simulink model "niof_model"  (R2021a)
settings: Solver=ode23tb  StartTime=0.0  StopTime=2  RelTol=1e-3
values from neighbouring files (symbols this model uses):
  h0 = ds.DateTime(1).Hour + ds.DateTime(1).Minute/60    [compiler_niof_model.m]
  S_area_hole = 0.01    [set_params_blocks.m]
undefined symbols (not defined in the file or in its folder): crop_GH1_NFT_slot1___C, crop_GH1_NFT_slot1___N, crop_GH1_NFT_slot1___R, crop_GH1_NFT_slot2___C, crop_GH1_NFT_slot2___N, crop_GH1_NFT_slot2___R, crop_GH1_NFT_slot3___C, crop_GH1_NFT_slot3___N, crop_GH1_NFT_slot3___R, crop_GH1_NFT_slot4___C, crop_GH1_NFT_slot4___N, crop_GH1_NFT_slot4___R, crop_GH1_RF_slot1___C, crop_GH1_RF_slot1___N, crop_GH1_RF_slot1___R, crop_GH1_RF_slot2___C, crop_GH1_RF_slot2___N, crop_GH1_RF_slot2___R, crop_GH1_RF_slot3___C, crop_GH1_RF_slot3___N, crop_GH1_RF_slot3___R, crop_GH1_RF_slot4___C, crop_GH1_RF_slot4___N, crop_GH1_RF_slot4___R, crop_GH2_RF_slot1___C, crop_GH2_RF_slot1___N, crop_GH2_RF_slot1___R, crop_GH2_RF_slot2___C, crop_GH2_RF_slot2___N, crop_GH2_RF_slot2___R, crop_GH2_RF_slot3___C, crop_GH2_RF_slot3___N, crop_GH2_RF_slot3___R, crop_GH2_RF_slot4___C, crop_GH2_RF_slot4___N, crop_GH2_RF_slot4___R, crop_GH2_TRAD_slot1___C, crop_GH2_TRAD_slot1___N, crop_GH2_TRAD_slot1___R, crop_GH2_TRAD_slot2___C, crop_GH2_TRAD_slot2___N, crop_GH2_TRAD_slot2___R, crop_GH2_TRAD_slot3___C, crop_GH2_TRAD_slot3___N, crop_GH2_TRAD_slot3___R, crop_GH2_TRAD_slot4___C, crop_GH2_TRAD_slot4___N, crop_GH2_TRAD_slot4___R, fish, GH3_Tank1_tend, GH3_Tank2_tend, GH3_Tank3_tend, GH3_Tank4_tend, tp_biofilter___T, tp_fish_C___T, tp_fish_M___T, tp_fish_S___T, tp_fish_T___T, tp_GH1_bio___T, tp_GH1_NFT___T ... (+3)
libraries: HORTISIM x152
(part 3 of 4)

== system niof_model/GH1/NFT System/Control 1 ==
  Crop : Inport
  Prune Policy : HORTISIM/Horticulture/Controls/Prune Policy  SystemSampleTime=-1  VariantActivationTime=update diagram  Latency=0  AutoFrameSizeCalculation=off
      settings: SourceProductName=Horti Simulator
  Scalar2Bus Control Crop : HORTISIM/Other  Functions/Scalar2Bus Control Crop  SystemSampleTime=-1  VariantActivationTime=update diagram  Latency=0  AutoFrameSizeCalculation=off
      settings: SourceProductName=Horti Simulator
  Start/Stop Window : HORTISIM/Other  Functions/Start//Stop Window  tinit=GH1_NFTSystem_Control1_tinit  tend=GH1_NFTSystem_Control1_tend
      settings: SourceProductName=Horti Simulator
  CC : Outport
  wires:
  ? -> Scalar2Bus Control Crop/3
  Prune Policy/1 -> Scalar2Bus Control Crop/1
  ? -> Scalar2Bus Control Crop/2
  Scalar2Bus Control Crop/1 -> CC/1
  Start/Stop Window/1 -> Scalar2Bus Control Crop/4
  Crop/1 -> Prune Policy/1

== system niof_model/GH1/NFT System/Control 2 ==
  Crop : Inport
  Prune Policy : HORTISIM/Horticulture/Controls/Prune Policy  SystemSampleTime=-1  VariantActivationTime=update diagram  Latency=0  AutoFrameSizeCalculation=off
      settings: SourceProductName=Horti Simulator
  Scalar2Bus Control Crop : HORTISIM/Other  Functions/Scalar2Bus Control Crop  SystemSampleTime=-1  VariantActivationTime=update diagram  Latency=0  AutoFrameSizeCalculation=off
      settings: SourceProductName=Horti Simulator
  Start/Stop Window : HORTISIM/Other  Functions/Start//Stop Window  tinit=GH1_NFTSystem_Control2_tinit  tend=GH1_NFTSystem_Control2_tend
      settings: SourceProductName=Horti Simulator
  CC : Outport
  wires:
  ? -> Scalar2Bus Control Crop/3
  Prune Policy/1 -> Scalar2Bus Control Crop/1
  ? -> Scalar2Bus Control Crop/2
  Scalar2Bus Control Crop/1 -> CC/1
  Start/Stop Window/1 -> Scalar2Bus Control Crop/4
  Crop/1 -> Prune Policy/1

== system niof_model/GH1/NFT System/Control 3 ==
  Crop : Inport
  Prune Policy : HORTISIM/Horticulture/Controls/Prune Policy  SystemSampleTime=-1  VariantActivationTime=update diagram  Latency=0  AutoFrameSizeCalculation=off
      settings: SourceProductName=Horti Simulator
  Scalar2Bus Control Crop : HORTISIM/Other  Functions/Scalar2Bus Control Crop  SystemSampleTime=-1  VariantActivationTime=update diagram  Latency=0  AutoFrameSizeCalculation=off
      settings: SourceProductName=Horti Simulator
  Start/Stop Window : HORTISIM/Other  Functions/Start//Stop Window  tinit=GH1_NFTSystem_Control3_tinit  tend=GH1_NFTSystem_Control3_tend
      settings: SourceProductName=Horti Simulator
  CC : Outport
  wires:
  ? -> Scalar2Bus Control Crop/3
  Prune Policy/1 -> Scalar2Bus Control Crop/1
  ? -> Scalar2Bus Control Crop/2
  Scalar2Bus Control Crop/1 -> CC/1
  Start/Stop Window/1 -> Scalar2Bus Control Crop/4
  Crop/1 -> Prune Policy/1

== system niof_model/GH1/NFT System/Control 4 ==
  Crop : Inport
  Prune Policy : HORTISIM/Horticulture/Controls/Prune Policy  SystemSampleTime=-1  VariantActivationTime=update diagram  Latency=0  AutoFrameSizeCalculation=off
      settings: SourceProductName=Horti Simulator
  Scalar2Bus Control Crop : HORTISIM/Other  Functions/Scalar2Bus Control Crop  SystemSampleTime=-1  VariantActivationTime=update diagram  Latency=0  AutoFrameSizeCalculation=off
      settings: SourceProductName=Horti Simulator
  Start/Stop Window : HORTISIM/Other  Functions/Start//Stop Window  tinit=GH1_NFTSystem_Control4_tinit  tend=GH1_NFTSystem_Control4_tend
      settings: SourceProductName=Horti Simulator
  CC : Outport
  wires:
  ? -> Scalar2Bus Control Crop/3
  Prune Policy/1 -> Scalar2Bus Control Crop/1
  ? -> Scalar2Bus Control Crop/2
  Scalar2Bus Control Crop/1 -> CC/1
  Start/Stop Window/1 -> Scalar2Bus Control Crop/4
  Crop/1 -> Prune Policy/1

== system niof_model/GH1/NFT System/Reorder signals ==
  In Bus Element : Inport  PortName=C1  Element=Crop
  In Bus Element1 : Inport  PortName=C1  Element=Crop1
  In Bus Element2 : Inport  PortName=C1  Element=Crop2
  In Bus Element3 : Inport  PortName=C1  Element=Crop3
  WT : Inport  Port=2
  Subsystem : Subsystem
      settings: PortSchema="{\"entries\":[{\"content\":{\"sides\":[{\"content\":{\"connectorIds\":[]},\"type\":\"ConnectorPlacement.EquallySpacedRectSide\",\"uuid\":\"331b7e07-99e0-48a1-afa9-efd959d86c3c\"},{\"content\":{\"connectorIds\":[\"Out1\",\"Out2\"],\"side\":\"RIGHT\"},\"type\":\"ConnectorPlacement.EquallySpacedRectSide\",\"uuid\":\"88f560c2-c33d-415c-abbb-9cce13a50e34\"},{\"content\":{\"connectorIds\":[\"In1\",\"In2\",\"In3\",\"In4\"],\"side\":\"TOP\"},\"type\":\"ConnectorPlacement.EquallySpacedRectSide\",\"uuid\":\"5809bd20-6d1a-4a08-a3be-af6196f2651a\"},{\"content\":{\"connectorIds\":[],\"side\":\"BOTTOM\"},\"type\":\"ConnectorPlacement.EquallySpacedRectSide\",\"uuid\":\"0451beb0-e3d9-4028-a291-a4662efcb901\"}]},\"type\":\"ConnectorPlacement.EquallySpacedConnector\",\"uuid\":\"8352e301-80a0-449c-83b8-038a5d79df4c\"}],\"packageUris\":[\"http://schema.mathworks.com/mf0/Connector/R2020b\"],\"version\":\"1.0\"}"
  Subsystem1 : Subsystem
      settings: PortSchema="{\"entries\":[{\"content\":{\"sides\":[{\"content\":{\"connectorIds\":[\"In1\",\"In2\",\"In3\",\"In4\"]},\"type\":\"ConnectorPlacement.EquallySpacedRectSide\",\"uuid\":\"4fbee580-d560-4e1c-bbb5-c1692f8814f1\"},{\"content\":{\"connectorIds\":[\"Out1\",\"Out2\",\"Out3\",\"Out4\"],\"side\":\"RIGHT\"},\"type\":\"ConnectorPlacement.EquallySpacedRectSide\",\"uuid\":\"81a4a23d-0981-460c-8110-0a6c3dae9561\"},{\"content\":{\"connectorIds\":[\"In5\"],\"side\":\"TOP\"},\"type\":\"ConnectorPlacement.EquallySpacedRectSide\",\"uuid\":\"d86bf355-ad16-490c-942f-99534b60638b\"},{\"content\":{\"connectorIds\":[\"Out5\"],\"side\":\"BOTTOM\"},\"type\":\"ConnectorPlacement.EquallySpacedRectSide\",\"uuid\":\"eaa009ab-e9b5-48b4-8c60-43d182c3bfd7\"}]},\"type\":\"ConnectorPlacement.EquallySpacedConnector\",\"uuid\":\"d99c9aa8-04cd-4090-9f71-30da2befe22b\"}],\"packageUris\":[\"http://schema.mathworks.com/mf0/Connector/R2020b\"],\"version\":\"1.0\"}"
  Out Bus Element : Outport  PortName=Subs  Element=Subs1
  Out Bus Element1 : Outport  PortName=Subs  Element=Subs2
  Out Bus Element2 : Outport  PortName=Subs  Element=Subs3
  Out Bus Element3 : Outport  PortName=Subs  Element=Subs4
  CropInt : Outport  Port=2
  fout : Outport  Port=3
  R : Outport  Port=4
  wires:
  WT/1 -> Subsystem1/5(WT)
  Subsystem1/4(Subs4) -> Out Bus Element3/1
  In Bus Element2/1 -> Subsystem/3(Crop2), Subsystem1/2(C2)
  Subsystem1/3(Subs3) -> Out Bus Element2/1
  In Bus Element/1 -> Subsystem1/1(C1), Subsystem/4(Crop1)
  Subsystem1/1(Subs) -> Out Bus Element/1
  Subsystem1/2(Subs2) -> Out Bus Element1/1
  Subsystem/2(Out2) -> R/1
  In Bus Element3/1 -> Subsystem1/3(C3), Subsystem/1(Crop3)
  Subsystem/1(Out1) -> fout/1
  In Bus Element1/1 -> Subsystem1/4(C4), Subsystem/2(Crop4)
  Subsystem1/5(Out3) -> CropInt/1

== system niof_model/GH1/RF System/Control 1 ==
  Crop : Inport
  Prune Policy : HORTISIM/Horticulture/Controls/Prune Policy  SystemSampleTime=-1  VariantActivationTime=update diagram  Latency=0  AutoFrameSizeCalculation=off
      settings: SourceProductName=Horti Simulator
  Scalar2Bus Control Crop : HORTISIM/Other  Functions/Scalar2Bus Control Crop  SystemSampleTime=-1  VariantActivationTime=update diagram  Latency=0  AutoFrameSizeCalculation=off
      settings: SourceProductName=Horti Simulator
  Start/Stop Window : HORTISIM/Other  Functions/Start//Stop Window  tinit=GH1_RFSystem_Control1_tinit  tend=GH1_RFSystem_Control1_tend
      settings: SourceProductName=Horti Simulator
  CC : Outport
  wires:
  ? -> Scalar2Bus Control Crop/3
  Prune Policy/1 -> Scalar2Bus Control Crop/1
  ? -> Scalar2Bus Control Crop/2
  Scalar2Bus Control Crop/1 -> CC/1
  Start/Stop Window/1 -> Scalar2Bus Control Crop/4
  Crop/1 -> Prune Policy/1

== system niof_model/GH1/RF System/Control 2 ==
  Crop : Inport
  Prune Policy : HORTISIM/Horticulture/Controls/Prune Policy  SystemSampleTime=-1  VariantActivationTime=update diagram  Latency=0  AutoFrameSizeCalculation=off
      settings: SourceProductName=Horti Simulator
  Scalar2Bus Control Crop : HORTISIM/Other  Functions/Scalar2Bus Control Crop  SystemSampleTime=-1  VariantActivationTime=update diagram  Latency=0  AutoFrameSizeCalculation=off
      settings: SourceProductName=Horti Simulator
  Start/Stop Window : HORTISIM/Other  Functions/Start//Stop Window  tinit=GH1_RFSystem_Control2_tinit  tend=GH1_RFSystem_Control2_tend
      settings: SourceProductName=Horti Simulator
  CC : Outport
  wires:
  ? -> Scalar2Bus Control Crop/3
  Prune Policy/1 -> Scalar2Bus Control Crop/1
  ? -> Scalar2Bus Control Crop/2
  Scalar2Bus Control Crop/1 -> CC/1
  Start/Stop Window/1 -> Scalar2Bus Control Crop/4
  Crop/1 -> Prune Policy/1

== system niof_model/GH1/RF System/Control 3 ==
  Crop : Inport
  Prune Policy : HORTISIM/Horticulture/Controls/Prune Policy  SystemSampleTime=-1  VariantActivationTime=update diagram  Latency=0  AutoFrameSizeCalculation=off
      settings: SourceProductName=Horti Simulator
  Scalar2Bus Control Crop : HORTISIM/Other  Functions/Scalar2Bus Control Crop  SystemSampleTime=-1  VariantActivationTime=update diagram  Latency=0  AutoFrameSizeCalculation=off
      settings: SourceProductName=Horti Simulator
  Start/Stop Window : HORTISIM/Other  Functions/Start//Stop Window  tinit=GH1_RFSystem_Control3_tinit  tend=GH1_RFSystem_Control3_tend
      settings: SourceProductName=Horti Simulator
  CC : Outport
  wires:
  ? -> Scalar2Bus Control Crop/3
  Prune Policy/1 -> Scalar2Bus Control Crop/1
  ? -> Scalar2Bus Control Crop/2
  Scalar2Bus Control Crop/1 -> CC/1
  Start/Stop Window/1 -> Scalar2Bus Control Crop/4
  Crop/1 -> Prune Policy/1

== system niof_model/GH1/RF System/Control 4 ==
  Crop : Inport
  Prune Policy : HORTISIM/Horticulture/Controls/Prune Policy  SystemSampleTime=-1  VariantActivationTime=update diagram  Latency=0  AutoFrameSizeCalculation=off
      settings: SourceProductName=Horti Simulator
  Scalar2Bus Control Crop : HORTISIM/Other  Functions/Scalar2Bus Control Crop  SystemSampleTime=-1  VariantActivationTime=update diagram  Latency=0  AutoFrameSizeCalculation=off
      settings: SourceProductName=Horti Simulator
  Start/Stop Window : HORTISIM/Other  Functions/Start//Stop Window  tinit=GH1_RFSystem_Control4_tinit  tend=GH1_RFSystem_Control4_tend
      settings: SourceProductName=Horti Simulator
  CC : Outport
  wires:
  ? -> Scalar2Bus Control Crop/3
  Prune Policy/1 -> Scalar2Bus Control Crop/1
  ? -> Scalar2Bus Control Crop/2
  Scalar2Bus Control Crop/1 -> CC/1
  Start/Stop Window/1 -> Scalar2Bus Control Crop/4
  Crop/1 -> Prune Policy/1

== system niof_model/GH1/RF System/Subsystem ==
  Crop2 : Inport
  Crop1 : Inport  Port=2
  Crop3 : Inport  Port=3
  Crop4 : Inport  Port=4
  CropToTank Parser{1..4} (4 alike) : HORTISIM/Other  Functions/CropToTank Parser  SystemSampleTime=-1  VariantActivationTime=update diagram  Latency=0  AutoFrameSizeCalculation=off
      settings: SourceProductName=Horti Simulator
  Vector Concatenate : Concatenate  NumInputs=4  Mode=Multidimensional array
  Vector Concatenate1 : Concatenate  NumInputs=4  Mode=Multidimensional array  ConcatenateDimension=2
  Out1 : Outport
  Out2 : Outport  Port=2
  wires:
  Crop2/1 -> CropToTank Parser2/1
  CropToTank Parser2/2 -> Vector Concatenate1/2
  CropToTank Parser1/2 -> Vector Concatenate1/1
  Vector Concatenate1/1 -> Out2/1
  Vector Concatenate/1 -> Out1/1
  Crop1/1 -> CropToTank Parser1/1
  CropToTank Parser2/1 -> Vector Concatenate/2
  CropToTank Parser1/1 -> Vector Concatenate/1
  Crop3/1 -> CropToTank Parser3/1
  CropToTank Parser3/1 -> Vector Concatenate/3
  Crop4/1 -> CropToTank Parser4/1
  CropToTank Parser4/1 -> Vector Concatenate/4
  CropToTank Parser3/2 -> Vector Concatenate1/3
  CropToTank Parser4/2 -> Vector Concatenate1/4

== system niof_model/GH1/RF System/Subsystem1 ==
  In Bus Element : Inport  PortName=C1  Element=Crop
  In Bus Element1 : Inport  PortName=C1  Element=Crop1
  In Bus Element2 : Inport  PortName=C1  Element=Crop2
  In Bus Element3 : Inport  PortName=C1  Element=Crop3
  WT : Inport  Port=2
  Crop Interactio with Climate : Subsystem
  TankToCrop Parser Several : Subsystem
      settings: PortSchema="{\"entries\":[{\"content\":{\"sides\":[{\"content\":{\"connectorIds\":[\"In1\",\"In2\",\"In3\",\"In4\"]},\"type\":\"ConnectorPlacement.EquallySpacedRectSide\",\"uuid\":\"99f6f79d-93b3-4d94-9532-d82544948055\"},{\"content\":{\"connectorIds\":[\"Out1\",\"Out2\",\"Out3\",\"Out4\"],\"side\":\"RIGHT\"},\"type\":\"ConnectorPlacement.EquallySpacedRectSide\",\"uuid\":\"ca15eaf2-1366-4114-b322-5e88a02c6d72\"},{\"content\":{\"connectorIds\":[\"In5\"],\"side\":\"TOP\"},\"type\":\"ConnectorPlacement.EquallySpacedRectSide\",\"uuid\":\"2404a174-e0a1-432d-a5bc-62127522feaf\"}]},\"type\":\"ConnectorPlacement.EquallySpacedConnector\",\"uuid\":\"a404298f-e4a9-4dc3-b790-516f41057283\"}],\"packageUris\":[\"http://schema.mathworks.com/mf0/Connector/R2020b\"],\"version\":\"1.0\"}"
  Subs1 : Outport
  Subs2 : Outport  Port=2
  Subs3 : Outport  Port=3
  Subs4 : Outport  Port=4
  Out3 : Outport  Port=5
  wires:
  Crop Interactio with Climate/1(OutBus) -> Out3/1
  WT/1 -> TankToCrop Parser Several/5(WT)
  TankToCrop Parser Several/1(Subs1) -> Subs1/1
  In Bus Element3/1 -> Crop Interactio with Climate/4(C4), TankToCrop Parser Several/4(C4)
  TankToCrop Parser Several/3(Subs3) -> Subs3/1
  TankToCrop Parser Several/4(Subs4) -> Subs4/1
  TankToCrop Parser Several/2(Subs2) -> Subs2/1
  In Bus Element2/1 -> Crop Interactio with Climate/3(C3), TankToCrop Parser Several/3(C3)
  In Bus Element/1 -> Crop Interactio with Climate/1(C1), TankToCrop Parser Several/1(C1)
  In Bus Element1/1 -> Crop Interactio with Climate/2(C2), TankToCrop Parser Several/2(C2)

== system niof_model/GH1/Subsystem1/Subsystem3 ==
  In1 : Inport
  In2 : Inport  Port=2
  Abs : Abs  ZeroCross=off
  Bus Creator : BusCreator  Inputs=3  OutDataTypeStr=Bus: FLOW  NonVirtualBus=on
  Bus Selector : BusSelector  OutputSignals=f
  Bus Selector1 : BusSelector  OutputSignals=f
  If : If  IfExpression=u1 <1e-8  ZeroCross=off
  If Action Subsystem : Subsystem  TreatAsAtomicUnit=on
  If Action Subsystem1 : Subsystem  TreatAsAtomicUnit=on
  Merge : Merge
  Merge1 : Merge
  Merge2 : Merge
  Sum : Sum  Inputs=|++
  Out1 : Outport
  wires:
  In1/1 -> [F1], Bus Selector/1
  In2/1 -> [F2], Bus Selector1/1
  Bus Selector/1 -> [f1]  "<f>"
  Bus Selector1/1 -> [f2]  "<f>"
  [f1] -> Sum/1
  [f2] -> Sum/2
  Sum/1 -> Abs/1
  Abs/1 -> If/1
  If/1 -> If Action Subsystem/Action
  [F1] -> If Action Subsystem/1(In1)
  [F2] -> If Action Subsystem1/2(In2)
  [F1] -> If Action Subsystem1/1(In1)
  Bus Creator/1 -> Out1/1
  If Action Subsystem1/3(X) -> Merge2/2
  If Action Subsystem/3(X) -> Merge2/1
  If Action Subsystem1/2(T) -> Merge1/2
  If Action Subsystem/2(T) -> Merge1/1
  If Action Subsystem1/1(f) -> Merge/2
  If Action Subsystem/1(f) -> Merge/1
  Merge/1 -> Bus Creator/1  "f"
  Merge1/1 -> Bus Creator/2  "T"
  Merge2/1 -> Bus Creator/3  "X"
  If/2 -> If Action Subsystem1/Action

== system niof_model/GH2/Mezcla Calor, Vapor de agua y CO2 desde los tanques de agua y la plantación/Crop2ExtArray ==
  In1 : Inport
  Bus Selector : BusSelector  OutputSignals=HeatVars.QV,HeatVars.QT,A_v,CC
  Scope : Scope
  Vector Concatenate : Concatenate  NumInputs=4  Mode=Multidimensional array
  Out1 : Outport
  wires:
  Vector Concatenate/1 -> Out1/1
  Bus Selector/4 -> Vector Concatenate/4  "<CC>"
  Bus Selector/3 -> Vector Concatenate/3  "<A_v>"
  Bus Selector/2 -> Scope/1, Vector Concatenate/2  "<QT>"
  Bus Selector/1 -> Vector Concatenate/1  "<QV>"
  In1/1 -> Bus Selector/1

== system niof_model/GH2/Mezcla Calor, Vapor de agua y CO2 desde los tanques de agua y la plantación/MatrixExt2Bus ==
  In1 : Inport
  Demux : Demux
  "Scalar2Bus Ext Signal " : HORTISIM/Other  Functions/Scalar2Bus Ext Signal    SystemSampleTime=-1  VariantActivationTime=update diagram  Latency=0  AutoFrameSizeCalculation=off
      settings: SourceProductName=Horti Simulator
  Scope : Scope
  Scope1 : Scope
  Sum of Elements : Sum  Inputs=+  CollapseMode=Specified dimension  CollapseDim=2
  CoCl : Outport
  wires:
  "Scalar2Bus Ext Signal "/1 -> CoCl/1
  Demux/4 -> "Scalar2Bus Ext Signal "/4
  Demux/3 -> Scope1/1, "Scalar2Bus Ext Signal "/3
  Demux/2 -> Scope/1, "Scalar2Bus Ext Signal "/2
  Demux/1 -> "Scalar2Bus Ext Signal "/1
  Sum of Elements/1 -> Demux/1
  In1/1 -> Sum of Elements/1

== system niof_model/GH2/Mezcla Calor, Vapor de agua y CO2 desde los tanques de agua y la plantación/Tank2ExtArray ==
  In1 : Inport
  Bus Selector : BusSelector  OutputSignals=QV,QT,A_t
  Constant : Constant  Value=0
  Scope : Scope
  Vector Concatenate : Concatenate  NumInputs=4  Mode=Multidimensional array
  Out1 : Outport
  wires:
  Vector Concatenate/1 -> Out1/1
  Constant/1 -> Vector Concatenate/4  "<CC>"
  Bus Selector/3 -> Vector Concatenate/3  "<A_t>"
  Bus Selector/2 -> Scope/1, Vector Concatenate/2  "<QT>"
  Bus Selector/1 -> Vector Concatenate/1  "<QV>"
  In1/1 -> Bus Selector/1

== system niof_model/GH2/RF System/Control 1 ==
  Crop : Inport
  Prune Policy : HORTISIM/Horticulture/Controls/Prune Policy  SystemSampleTime=-1  VariantActivationTime=update diagram  Latency=0  AutoFrameSizeCalculation=off
      settings: SourceProductName=Horti Simulator
  Scalar2Bus Control Crop : HORTISIM/Other  Functions/Scalar2Bus Control Crop  SystemSampleTime=-1  VariantActivationTime=update diagram  Latency=0  AutoFrameSizeCalculation=off
      settings: SourceProductName=Horti Simulator
  Start/Stop Window : HORTISIM/Other  Functions/Start//Stop Window  tinit=GH2_RFSystem_Control1_tinit  tend=GH2_RFSystem_Control1_tend
      settings: SourceProductName=Horti Simulator
  CC : Outport
  wires:
  ? -> Scalar2Bus Control Crop/3
  Prune Policy/1 -> Scalar2Bus Control Crop/1
  ? -> Scalar2Bus Control Crop/2
  Scalar2Bus Control Crop/1 -> CC/1
  Start/Stop Window/1 -> Scalar2Bus Control Crop/4
  Crop/1 -> Prune Policy/1

== system niof_model/GH2/RF System/Control 2 ==
  Crop : Inport
  Prune Policy : HORTISIM/Horticulture/Controls/Prune Policy  SystemSampleTime=-1  VariantActivationTime=update diagram  Latency=0  AutoFrameSizeCalculation=off
      settings: SourceProductName=Horti Simulator
  Scalar2Bus Control Crop : HORTISIM/Other  Functions/Scalar2Bus Control Crop  SystemSampleTime=-1  VariantActivationTime=update diagram  Latency=0  AutoFrameSizeCalculation=off
      settings: SourceProductName=Horti Simulator
  Start/Stop Window : HORTISIM/Other  Functions/Start//Stop Window  tinit=GH2_RFSystem_Control2_tinit  tend=GH2_RFSystem_Control2_tend
      settings: SourceProductName=Horti Simulator
  CC : Outport
  wires:
  ? -> Scalar2Bus Control Crop/3
  Prune Policy/1 -> Scalar2Bus Control Crop/1
  ? -> Scalar2Bus Control Crop/2
  Scalar2Bus Control Crop/1 -> CC/1
  Start/Stop Window/1 -> Scalar2Bus Control Crop/4
  Crop/1 -> Prune Policy/1

== system niof_model/GH2/RF System/Control 3 ==
  Crop : Inport
  Prune Policy : HORTISIM/Horticulture/Controls/Prune Policy  SystemSampleTime=-1  VariantActivationTime=update diagram  Latency=0  AutoFrameSizeCalculation=off
      settings: SourceProductName=Horti Simulator
  Scalar2Bus Control Crop : HORTISIM/Other  Functions/Scalar2Bus Control Crop  SystemSampleTime=-1  VariantActivationTime=update diagram  Latency=0  AutoFrameSizeCalculation=off
      settings: SourceProductName=Horti Simulator
  Start/Stop Window : HORTISIM/Other  Functions/Start//Stop Window  tinit=GH2_RFSystem_Control3_tinit  tend=GH2_RFSystem_Control3_tend
      settings: SourceProductName=Horti Simulator
  CC : Outport
  wires:
  ? -> Scalar2Bus Control Crop/3
  Prune Policy/1 -> Scalar2Bus Control Crop/1
  ? -> Scalar2Bus Control Crop/2
  Scalar2Bus Control Crop/1 -> CC/1
  Start/Stop Window/1 -> Scalar2Bus Control Crop/4
  Crop/1 -> Prune Policy/1

== system niof_model/GH2/RF System/Control 4 ==
  Crop : Inport
  Prune Policy : HORTISIM/Horticulture/Controls/Prune Policy  SystemSampleTime=-1  VariantActivationTime=update diagram  Latency=0  AutoFrameSizeCalculation=off
      settings: SourceProductName=Horti Simulator
  Scalar2Bus Control Crop : HORTISIM/Other  Functions/Scalar2Bus Control Crop  SystemSampleTime=-1  VariantActivationTime=update diagram  Latency=0  AutoFrameSizeCalculation=off
      settings: SourceProductName=Horti Simulator
  Start/Stop Window : HORTISIM/Other  Functions/Start//Stop Window  tinit=GH2_RFSystem_Control4_tinit  tend=GH2_RFSystem_Control4_tend
      settings: SourceProductName=Horti Simulator
  CC : Outport
  wires:
  ? -> Scalar2Bus Control Crop/3
  Prune Policy/1 -> Scalar2Bus Control Crop/1
  ? -> Scalar2Bus Control Crop/2
  Scalar2Bus Control Crop/1 -> CC/1
  Start/Stop Window/1 -> Scalar2Bus Control Crop/4
  Crop/1 -> Prune Policy/1

== system niof_model/GH2/RF System/Subsystem ==
  Crop2 : Inport
  Crop1 : Inport  Port=2
  Crop3 : Inport  Port=3
  Crop4 : Inport  Port=4
  CropToTank Parser{1..4} (4 alike) : HORTISIM/Other  Functions/CropToTank Parser  SystemSampleTime=-1  VariantActivationTime=update diagram  Latency=0  AutoFrameSizeCalculation=off
      settings: SourceProductName=Horti Simulator
  Vector Concatenate : Concatenate  NumInputs=4  Mode=Multidimensional array
  Vector Concatenate1 : Concatenate  NumInputs=4  Mode=Multidimensional array  ConcatenateDimension=2
  Out1 : Outport
  Out2 : Outport  Port=2
  wires:
  Crop2/1 -> CropToTank Parser2/1
  CropToTank Parser2/2 -> Vector Concatenate1/2
  CropToTank Parser1/2 -> Vector Concatenate1/1
  Vector Concatenate1/1 -> Out2/1
  Vector Concatenate/1 -> Out1/1
  Crop1/1 -> CropToTank Parser1/1
  CropToTank Parser2/1 -> Vector Concatenate/2
  CropToTank Parser1/1 -> Vector Concatenate/1
  Crop3/1 -> CropToTank Parser3/1
  CropToTank Parser3/1 -> Vector Concatenate/3
  Crop4/1 -> CropToTank Parser4/1
  CropToTank Parser4/1 -> Vector Concatenate/4
  CropToTank Parser3/2 -> Vector Concatenate1/3
  CropToTank Parser4/2 -> Vector Concatenate1/4

== system niof_model/GH2/RF System/Subsystem1 ==
  In Bus Element : Inport  PortName=C1  Element=Crop
  In Bus Element1 : Inport  PortName=C1  Element=Crop1
  In Bus Element2 : Inport  PortName=C1  Element=Crop2
  In Bus Element3 : Inport  PortName=C1  Element=Crop3
  WT : Inport  Port=2
  Crop Interactio with Climate : Subsystem
  TankToCrop Parser Several : Subsystem
      settings: PortSchema="{\"entries\":[{\"content\":{\"sides\":[{\"content\":{\"connectorIds\":[\"In1\",\"In2\",\"In3\",\"In4\"]},\"type\":\"ConnectorPlacement.EquallySpacedRectSide\",\"uuid\":\"99f6f79d-93b3-4d94-9532-d82544948055\"},{\"content\":{\"connectorIds\":[\"Out1\",\"Out2\",\"Out3\",\"Out4\"],\"side\":\"RIGHT\"},\"type\":\"ConnectorPlacement.EquallySpacedRectSide\",\"uuid\":\"ca15eaf2-1366-4114-b322-5e88a02c6d72\"},{\"content\":{\"connectorIds\":[\"In5\"],\"side\":\"TOP\"},\"type\":\"ConnectorPlacement.EquallySpacedRectSide\",\"uuid\":\"2404a174-e0a1-432d-a5bc-62127522feaf\"}]},\"type\":\"ConnectorPlacement.EquallySpacedConnector\",\"uuid\":\"a404298f-e4a9-4dc3-b790-516f41057283\"}],\"packageUris\":[\"http://schema.mathworks.com/mf0/Connector/R2020b\"],\"version\":\"1.0\"}"
  Subs1 : Outport
  Subs2 : Outport  Port=2
  Subs3 : Outport  Port=3
  Subs4 : Outport  Port=4
  Out3 : Outport  Port=5
  wires:
  Crop Interactio with Climate/1(OutBus) -> Out3/1
  WT/1 -> TankToCrop Parser Several/5(WT)
  TankToCrop Parser Several/1(Subs1) -> Subs1/1
  In Bus Element3/1 -> Crop Interactio with Climate/4(C4), TankToCrop Parser Several/4(C4)
  TankToCrop Parser Several/3(Subs3) -> Subs3/1
  TankToCrop Parser Several/4(Subs4) -> Subs4/1
  TankToCrop Parser Several/2(Subs2) -> Subs2/1
  In Bus Element2/1 -> Crop Interactio with Climate/3(C3), TankToCrop Parser Several/3(C3)
  In Bus Element/1 -> Crop Interactio with Climate/1(C1), TankToCrop Parser Several/1(C1)
  In Bus Element1/1 -> Crop Interactio with Climate/2(C2), TankToCrop Parser Several/2(C2)

== system niof_model/GH2/TRAD System/Control 1 ==
  Crop : Inport
  Prune Policy : HORTISIM/Horticulture/Controls/Prune Policy  SystemSampleTime=-1  VariantActivationTime=update diagram  Latency=0  AutoFrameSizeCalculation=off
      settings: SourceProductName=Horti Simulator
  Scalar2Bus Control Crop : HORTISIM/Other  Functions/Scalar2Bus Control Crop  SystemSampleTime=-1  VariantActivationTime=update diagram  Latency=0  AutoFrameSizeCalculation=off
      settings: SourceProductName=Horti Simulator
  Start/Stop Window : HORTISIM/Other  Functions/Start//Stop Window  tinit=GH2_TRADSystem_Control1_tinit  tend=GH2_TRADSystem_Control1_tend
      settings: SourceProductName=Horti Simulator
  CC : Outport
  wires:
  ? -> Scalar2Bus Control Crop/3
  Prune Policy/1 -> Scalar2Bus Control Crop/1
  ? -> Scalar2Bus Control Crop/2
  Scalar2Bus Control Crop/1 -> CC/1
  Start/Stop Window/1 -> Scalar2Bus Control Crop/4
  Crop/1 -> Prune Policy/1

== system niof_model/GH2/TRAD System/Control 2 ==
  Crop : Inport
  Prune Policy : HORTISIM/Horticulture/Controls/Prune Policy  SystemSampleTime=-1  VariantActivationTime=update diagram  Latency=0  AutoFrameSizeCalculation=off
      settings: SourceProductName=Horti Simulator
  Scalar2Bus Control Crop : HORTISIM/Other  Functions/Scalar2Bus Control Crop  SystemSampleTime=-1  VariantActivationTime=update diagram  Latency=0  AutoFrameSizeCalculation=off
      settings: SourceProductName=Horti Simulator
  Start/Stop Window : HORTISIM/Other  Functions/Start//Stop Window  tinit=GH2_TRADSystem_Control2_tinit  tend=GH2_TRADSystem_Control2_tend
      settings: SourceProductName=Horti Simulator
  CC : Outport
  wires:
  ? -> Scalar2Bus Control Crop/3
  Prune Policy/1 -> Scalar2Bus Control Crop/1
  ? -> Scalar2Bus Control Crop/2
  Scalar2Bus Control Crop/1 -> CC/1
  Start/Stop Window/1 -> Scalar2Bus Control Crop/4
  Crop/1 -> Prune Policy/1

== system niof_model/GH2/TRAD System/Control 3 ==
  Crop : Inport
  Prune Policy : HORTISIM/Horticulture/Controls/Prune Policy  SystemSampleTime=-1  VariantActivationTime=update diagram  Latency=0  AutoFrameSizeCalculation=off
      settings: SourceProductName=Horti Simulator
  Scalar2Bus Control Crop : HORTISIM/Other  Functions/Scalar2Bus Control Crop  SystemSampleTime=-1  VariantActivationTime=update diagram  Latency=0  AutoFrameSizeCalculation=off
      settings: SourceProductName=Horti Simulator
  Start/Stop Window : HORTISIM/Other  Functions/Start//Stop Window  tinit=GH2_TRADSystem_Control3_tinit  tend=GH2_TRADSystem_Control3_tend
      settings: SourceProductName=Horti Simulator
  CC : Outport
  wires:
  ? -> Scalar2Bus Control Crop/3
  Prune Policy/1 -> Scalar2Bus Control Crop/1
  ? -> Scalar2Bus Control Crop/2
  Scalar2Bus Control Crop/1 -> CC/1
  Start/Stop Window/1 -> Scalar2Bus Control Crop/4
  Crop/1 -> Prune Policy/1

== system niof_model/GH2/TRAD System/Control 4 ==
  Crop : Inport
  Prune Policy : HORTISIM/Horticulture/Controls/Prune Policy  SystemSampleTime=-1  VariantActivationTime=update diagram  Latency=0  AutoFrameSizeCalculation=off
      settings: SourceProductName=Horti Simulator
  Scalar2Bus Control Crop : HORTISIM/Other  Functions/Scalar2Bus Control Crop  SystemSampleTime=-1  VariantActivationTime=update diagram  Latency=0  AutoFrameSizeCalculation=off
      settings: SourceProductName=Horti Simulator
  Start/Stop Window : HORTISIM/Other  Functions/Start//Stop Window  tinit=GH2_TRADSystem_Control4_tinit  tend=GH2_TRADSystem_Control4_tend
      settings: SourceProductName=Horti Simulator
  CC : Outport
  wires:
  ? -> Scalar2Bus Control Crop/3
  Prune Policy/1 -> Scalar2Bus Control Crop/1
  ? -> Scalar2Bus Control Crop/2
  Scalar2Bus Control Crop/1 -> CC/1
  Start/Stop Window/1 -> Scalar2Bus Control Crop/4
  Crop/1 -> Prune Policy/1

== system niof_model/GH2/TRAD System/Subsystem ==
  Crop2 : Inport
  Crop1 : Inport  Port=2
  Crop3 : Inport  Port=3
  Crop4 : Inport  Port=4
  CropToTank Parser{1..4} (4 alike) : HORTISIM/Other  Functions/CropToTank Parser  SystemSampleTime=-1  VariantActivationTime=update diagram  Latency=0  AutoFrameSizeCalculation=off
      settings: SourceProductName=Horti Simulator
  Vector Concatenate : Concatenate  NumInputs=4  Mode=Multidimensional array
  Vector Concatenate1 : Concatenate  NumInputs=4  Mode=Multidimensional array  ConcatenateDimension=2
  Out1 : Outport
  Out2 : Outport  Port=2
  wires:
  Crop2/1 -> CropToTank Parser2/1
  CropToTank Parser2/2 -> Vector Concatenate1/2
  CropToTank Parser1/2 -> Vector Concatenate1/1
  Vector Concatenate1/1 -> Out2/1
  Vector Concatenate/1 -> Out1/1
  Crop1/1 -> CropToTank Parser1/1
  CropToTank Parser2/1 -> Vector Concatenate/2
  CropToTank Parser1/1 -> Vector Concatenate/1
  Crop3/1 -> CropToTank Parser3/1
  CropToTank Parser3/1 -> Vector Concatenate/3
  Crop4/1 -> CropToTank Parser4/1
  CropToTank Parser4/1 -> Vector Concatenate/4
  CropToTank Parser3/2 -> Vector Concatenate1/3
  CropToTank Parser4/2 -> Vector Concatenate1/4

== system niof_model/GH2/TRAD System/Subsystem1 ==
  In Bus Element : Inport  PortName=C1  Element=Crop
  In Bus Element1 : Inport  PortName=C1  Element=Crop1
  In Bus Element2 : Inport  PortName=C1  Element=Crop2
  In Bus Element3 : Inport  PortName=C1  Element=Crop3
  WT : Inport  Port=2
  Crop Interactio with Climate : Subsystem
  TankToCrop Parser Several : Subsystem
      settings: PortSchema="{\"entries\":[{\"content\":{\"sides\":[{\"content\":{\"connectorIds\":[\"In1\",\"In2\",\"In3\",\"In4\"]},\"type\":\"ConnectorPlacement.EquallySpacedRectSide\",\"uuid\":\"99f6f79d-93b3-4d94-9532-d82544948055\"},{\"content\":{\"connectorIds\":[\"Out1\",\"Out2\",\"Out3\",\"Out4\"],\"side\":\"RIGHT\"},\"type\":\"ConnectorPlacement.EquallySpacedRectSide\",\"uuid\":\"ca15eaf2-1366-4114-b322-5e88a02c6d72\"},{\"content\":{\"connectorIds\":[\"In5\"],\"side\":\"TOP\"},\"type\":\"ConnectorPlacement.EquallySpacedRectSide\",\"uuid\":\"2404a174-e0a1-432d-a5bc-62127522feaf\"}]},\"type\":\"ConnectorPlacement.EquallySpacedConnector\",\"uuid\":\"a404298f-e4a9-4dc3-b790-516f41057283\"}],\"packageUris\":[\"http://schema.mathworks.com/mf0/Connector/R2020b\"],\"version\":\"1.0\"}"
  Subs1 : Outport
  Subs2 : Outport  Port=2
  Subs3 : Outport  Port=3
  Subs4 : Outport  Port=4
  Out3 : Outport  Port=5
  wires:
  Crop Interactio with Climate/1(OutBus) -> Out3/1
  WT/1 -> TankToCrop Parser Several/5(WT)
  TankToCrop Parser Several/1(Subs1) -> Subs1/1
  In Bus Element3/1 -> Crop Interactio with Climate/4(C4), TankToCrop Parser Several/4(C4)
  TankToCrop Parser Several/3(Subs3) -> Subs3/1
  TankToCrop Parser Several/4(Subs4) -> Subs4/1
  TankToCrop Parser Several/2(Subs2) -> Subs2/1
  In Bus Element2/1 -> Crop Interactio with Climate/3(C3), TankToCrop Parser Several/3(C3)
  In Bus Element/1 -> Crop Interactio with Climate/1(C1), TankToCrop Parser Several/1(C1)
  In Bus Element1/1 -> Crop Interactio with Climate/2(C2), TankToCrop Parser Several/2(C2)

== system niof_model/GH2/add drainge flows/If Action Subsystem ==
  In1 : Inport
  Action Port : ActionPort  ActionPortLabel=if(u1 <1e-8)
  Bus Selector : BusSelector  OutputSignals=f,T,X
  f : Outport
  T : Outport  Port=2
  X : Outport  Port=3
  wires:
  In1/1 -> Bus Selector/1
  Bus Selector/1 -> f/1  "<f>"
  Bus Selector/2 -> T/1  "<T>"
  Bus Selector/3 -> X/1  "<X>"

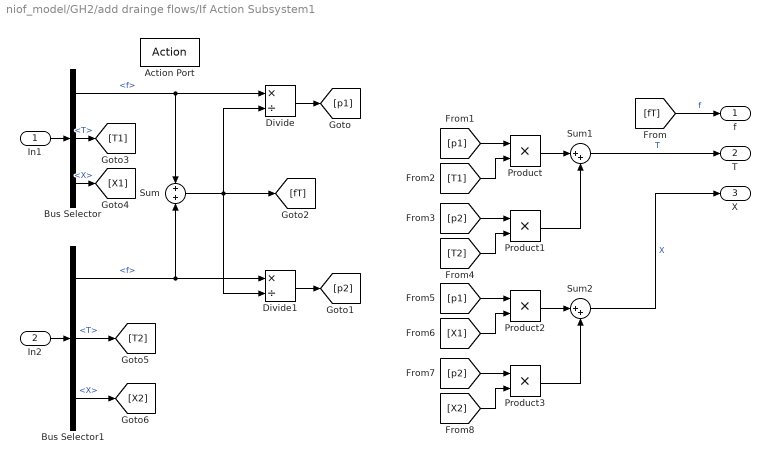
== system niof_model/GH2/add drainge flows/If Action Subsystem1 ==
  In1 : Inport
  In2 : Inport  Port=2
  Action Port : ActionPort  ActionPortLabel=else
  Bus Selector : BusSelector  OutputSignals=f,T,X
  Bus Selector1 : BusSelector  OutputSignals=f,T,X
  Divide : Product  Inputs=*/
  Divide1 : Product  Inputs=*/
  Product{,1..3} (4 alike) : Product
  Sum : Sum
  Sum1 : Sum  Inputs=|++
  Sum2 : Sum  Inputs=|++
  f : Outport
  T : Outport  Port=2
  X : Outport  Port=3
  wires:
  In1/1 -> Bus Selector/1
  In2/1 -> Bus Selector1/1
  Bus Selector/1 -> Sum/1, Divide/1  "<f>"
  Bus Selector1/1 -> Sum/2, Divide1/1  "<f>"
  Sum/1 -> Divide1/2, [fT], Divide/2
  Divide/1 -> [p1]
  Divide1/1 -> [p2]
  [fT] -> f/1  "f"
  Bus Selector/2 -> [T1]  "<T>"
  Bus Selector/3 -> [X1]  "<X>"
  Bus Selector1/2 -> [T2]  "<T>"
  Bus Selector1/3 -> [X2]  "<X>"
  [p1] -> Product/1
  [T1] -> Product/2
  [p2] -> Product1/1
  [T2] -> Product1/2
  Product/1 -> Sum1/1
  Product1/1 -> Sum1/2
  Sum1/1 -> T/1  "T"
  [p1] -> Product2/1
  [X2] -> Product3/2
  [p2] -> Product3/1
  Sum2/1 -> X/1  "X"
  Product3/1 -> Sum2/2
  Product2/1 -> Sum2/1
  [X1] -> Product2/2

== system niof_model/GH1/NFT System/Reorder signals/Subsystem ==
  Crop3 : Inport
  Crop4 : Inport  Port=2
  Crop2 : Inport  Port=3
  Crop1 : Inport  Port=4
  CropToTank Parser{1..4} (4 alike) : HORTISIM/Other  Functions/CropToTank Parser  SystemSampleTime=-1  VariantActivationTime=update diagram  Latency=0  AutoFrameSizeCalculation=off
      settings: SourceProductName=Horti Simulator
  Vector Concatenate : Concatenate  NumInputs=4  Mode=Multidimensional array
  Vector Concatenate1 : Concatenate  NumInputs=4  Mode=Multidimensional array  ConcatenateDimension=2
  Out1 : Outport
  Out2 : Outport  Port=2
  wires:
  Crop2/1 -> CropToTank Parser2/1
  CropToTank Parser2/2 -> Vector Concatenate1/2
  CropToTank Parser1/2 -> Vector Concatenate1/1
  Vector Concatenate1/1 -> Out2/1
  Vector Concatenate/1 -> Out1/1
  Crop1/1 -> CropToTank Parser1/1
  CropToTank Parser2/1 -> Vector Concatenate/2
  CropToTank Parser1/1 -> Vector Concatenate/1
  Crop3/1 -> CropToTank Parser3/1
  CropToTank Parser3/1 -> Vector Concatenate/3
  Crop4/1 -> CropToTank Parser4/1
  CropToTank Parser4/1 -> Vector Concatenate/4
  CropToTank Parser3/2 -> Vector Concatenate1/3
  CropToTank Parser4/2 -> Vector Concatenate1/4

== system niof_model/GH1/NFT System/Reorder signals/Subsystem1 ==
  C1 : Inport
  C2 : Inport  Port=2
  C3 : Inport  Port=3
  C4 : Inport  Port=4
  WT : Inport  Port=5
  Crop Interactio with Climate : Subsystem
  TankToCrop Parser Several : Subsystem
      settings: PortSchema="{\"entries\":[{\"content\":{\"sides\":[{\"content\":{\"connectorIds\":[\"In1\",\"In2\",\"In3\",\"In4\"]},\"type\":\"ConnectorPlacement.EquallySpacedRectSide\",\"uuid\":\"99f6f79d-93b3-4d94-9532-d82544948055\"},{\"content\":{\"connectorIds\":[\"Out1\",\"Out2\",\"Out3\",\"Out4\"],\"side\":\"RIGHT\"},\"type\":\"ConnectorPlacement.EquallySpacedRectSide\",\"uuid\":\"ca15eaf2-1366-4114-b322-5e88a02c6d72\"},{\"content\":{\"connectorIds\":[\"In5\"],\"side\":\"TOP\"},\"type\":\"ConnectorPlacement.EquallySpacedRectSide\",\"uuid\":\"2404a174-e0a1-432d-a5bc-62127522feaf\"}]},\"type\":\"ConnectorPlacement.EquallySpacedConnector\",\"uuid\":\"a404298f-e4a9-4dc3-b790-516f41057283\"}],\"packageUris\":[\"http://schema.mathworks.com/mf0/Connector/R2020b\"],\"version\":\"1.0\"}"
  Subs : Outport
  Subs2 : Outport  Port=2
  Subs3 : Outport  Port=3
  Subs4 : Outport  Port=4
  Out3 : Outport  Port=5
  wires:
  Crop Interactio with Climate/1(OutBus) -> Out3/1
  WT/1 -> TankToCrop Parser Several/5(WT)
  TankToCrop Parser Several/1(Subs1) -> Subs/1
  C4/1 -> Crop Interactio with Climate/4(C4), TankToCrop Parser Several/4(C4)
  TankToCrop Parser Several/3(Subs3) -> Subs3/1
  TankToCrop Parser Several/4(Subs4) -> Subs4/1
  TankToCrop Parser Several/2(Subs2) -> Subs2/1
  C3/1 -> Crop Interactio with Climate/3(C3), TankToCrop Parser Several/3(C3)
  C1/1 -> Crop Interactio with Climate/1(C1), TankToCrop Parser Several/1(C1)
  C2/1 -> Crop Interactio with Climate/2(C2), TankToCrop Parser Several/2(C2)

== system niof_model/GH1/RF System/Subsystem1/Crop Interactio with Climate ==
  C1 : Inport
  C2 : Inport  Port=2
  C3 : Inport  Port=3
  C4 : Inport  Port=4
  Crop2ExtArray{,1..3} (4 alike) : HORTISIM/Other  Functions/Crop2ExtArray  SystemSampleTime=-1  VariantActivationTime=update diagram  Latency=0  AutoFrameSizeCalculation=off
      settings: SourceProductName=Horti Simulator
  Demux : Demux
  Sum : Sum  Inputs=+  CollapseMode=Specified dimension  CollapseDim=2
  Vector Concatenate : Concatenate  NumInputs=4  Mode=Multidimensional array  ConcatenateDimension=2
  Out Bus Element : Outport  PortName=OutBus  Element=HeatVars.QV
  Out Bus Element1 : Outport  PortName=OutBus  Element=HeatVars.QT
  Out Bus Element2 : Outport  PortName=OutBus  Element=A_v
  Out Bus Element3 : Outport  PortName=OutBus  Element=CC
  wires:
  C1/1 -> Crop2ExtArray/1
  C2/1 -> Crop2ExtArray1/1
  C3/1 -> Crop2ExtArray2/1
  C4/1 -> Crop2ExtArray3/1
  Crop2ExtArray3/1 -> Vector Concatenate/4
  Crop2ExtArray2/1 -> Vector Concatenate/3
  Crop2ExtArray1/1 -> Vector Concatenate/2
  Crop2ExtArray/1 -> Vector Concatenate/1
  Vector Concatenate/1 -> Sum/1
  Sum/1 -> Demux/1
  Demux/1 -> Out Bus Element/1
  Demux/2 -> Out Bus Element1/1
  Demux/3 -> Out Bus Element2/1
  Demux/4 -> Out Bus Element3/1

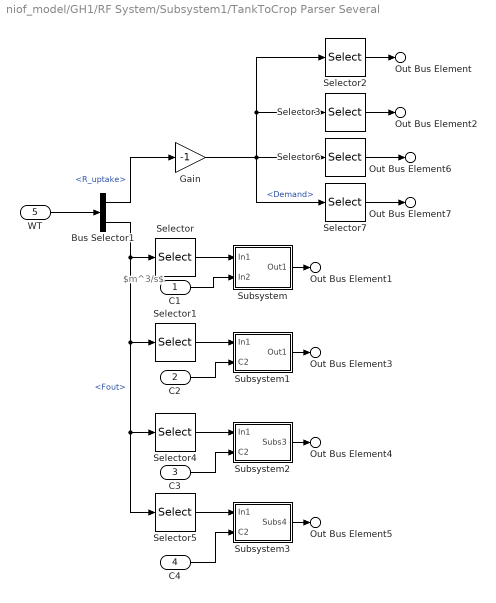
== system niof_model/GH1/RF System/Subsystem1/TankToCrop Parser Several ==
  note: $m^3/s$
  C1 : Inport
  C2 : Inport  Port=2
  C3 : Inport  Port=3
  C4 : Inport  Port=4
  WT : Inport  Port=5
  Bus Selector1 : BusSelector  OutputSignals=R_uptake,Fout
  Gain : Gain  Gain=-1
  Selector : Selector  InputPortWidth=4  IndexOptions=Index vector (dialog)  Indices=[1]  OutputSizes=1
  Selector1 : Selector  InputPortWidth=4  IndexOptions=Index vector (dialog)  Indices=[2]  OutputSizes=1
  Selector2 : Selector  NumberOfDimensions=2  InputPortWidth=2  IndexOptions=Select all,Index vector (dialog)  Indices=[1],1  OutputSizes=1,1
  Selector3 : Selector  NumberOfDimensions=2  InputPortWidth=2  IndexOptions=Select all,Index vector (dialog)  Indices=[2],2  OutputSizes=1,1
  Selector4 : Selector  InputPortWidth=4  IndexOptions=Index vector (dialog)  Indices=[3]  OutputSizes=1
  Selector5 : Selector  InputPortWidth=4  IndexOptions=Index vector (dialog)  Indices=[4]  OutputSizes=1
  Selector6 : Selector  NumberOfDimensions=2  InputPortWidth=2  IndexOptions=Select all,Index vector (dialog)  Indices=[2],3  OutputSizes=1,1
  Selector7 : Selector  NumberOfDimensions=2  InputPortWidth=2  IndexOptions=Select all,Index vector (dialog)  Indices=[2],4  OutputSizes=1,1
  Subsystem : Subsystem
  Subsystem1 : Subsystem
  Subsystem2 : Subsystem
  Subsystem3 : Subsystem
  Out Bus Element : Outport  PortName=Subs1  Element=Uptake.Nutrients
  Out Bus Element1 : Outport  PortName=Subs1  Element=Uptake.Water
  Out Bus Element2 : Outport  Port=2  PortName=Subs2  Element=Uptake.Nutrients
  Out Bus Element3 : Outport  Port=2  PortName=Subs2  Element=Uptake.Water
  Out Bus Element6 : Outport  Port=3  PortName=Subs3  Element=Uptake.Nutrients
  Out Bus Element4 : Outport  Port=3  PortName=Subs3  Element=Uptake.Water
  Out Bus Element7 : Outport  Port=4  PortName=Subs4  Element=Uptake.Nutrients
  Out Bus Element5 : Outport  Port=4  PortName=Subs4  Element=Uptake.Water
  wires:
  WT/1 -> Bus Selector1/1
  Bus Selector1/1 -> Gain/1  "<R_uptake>"
  Gain/1 -> Selector7/1, Selector6/1, Selector3/1, Selector2/1  "<Demand>"
  Selector2/1 -> Out Bus Element/1
  Selector3/1 -> Out Bus Element2/1
  Selector/1 -> Subsystem/1(In1)
  C1/1 -> Subsystem/2(In2)
  Subsystem/1(Out1) -> Out Bus Element1/1
  Selector1/1 -> Subsystem1/1(In1)
  C2/1 -> Subsystem1/2(C2)
  Subsystem1/1(Out1) -> Out Bus Element3/1
  Selector4/1 -> Subsystem2/1(In1)
  C3/1 -> Subsystem2/2(C2)
  Bus Selector1/2 -> Selector5/1, Selector4/1, Selector1/1, Selector/1  "<Fout>"
  Selector5/1 -> Subsystem3/1(In1)
  C4/1 -> Subsystem3/2(C2)
  Subsystem2/1("Subs3 ") -> Out Bus Element4/1
  Subsystem3/1(Subs4) -> Out Bus Element5/1
  Selector6/1 -> Out Bus Element6/1
  Selector7/1 -> Out Bus Element7/1

== system niof_model/GH1/Subsystem1/Subsystem3/If Action Subsystem ==
  In1 : Inport
  Action Port : ActionPort  ActionPortLabel=if(u1 <1e-8)
  Bus Selector : BusSelector  OutputSignals=f,T,X
  f : Outport
  T : Outport  Port=2
  X : Outport  Port=3
  wires:
  In1/1 -> Bus Selector/1
  Bus Selector/1 -> f/1  "<f>"
  Bus Selector/2 -> T/1  "<T>"
  Bus Selector/3 -> X/1  "<X>"

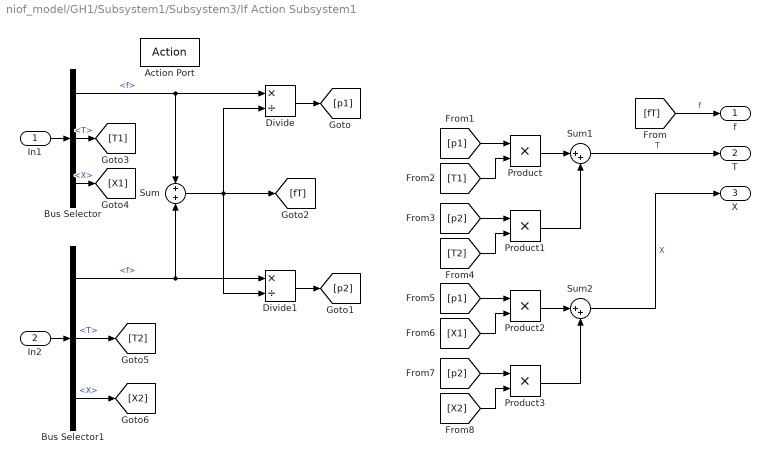
== system niof_model/GH1/Subsystem1/Subsystem3/If Action Subsystem1 ==
  In1 : Inport
  In2 : Inport  Port=2
  Action Port : ActionPort  ActionPortLabel=else
  Bus Selector : BusSelector  OutputSignals=f,T,X
  Bus Selector1 : BusSelector  OutputSignals=f,T,X
  Divide : Product  Inputs=*/
  Divide1 : Product  Inputs=*/
  Product{,1..3} (4 alike) : Product
  Sum : Sum
  Sum1 : Sum  Inputs=|++
  Sum2 : Sum  Inputs=|++
  f : Outport
  T : Outport  Port=2
  X : Outport  Port=3
  wires:
  In1/1 -> Bus Selector/1
  In2/1 -> Bus Selector1/1
  Bus Selector/1 -> Sum/1, Divide/1  "<f>"
  Bus Selector1/1 -> Sum/2, Divide1/1  "<f>"
  Sum/1 -> Divide1/2, [fT], Divide/2
  Divide/1 -> [p1]
  Divide1/1 -> [p2]
  [fT] -> f/1  "f"
  Bus Selector/2 -> [T1]  "<T>"
  Bus Selector/3 -> [X1]  "<X>"
  Bus Selector1/2 -> [T2]  "<T>"
  Bus Selector1/3 -> [X2]  "<X>"
  [p1] -> Product/1
  [T1] -> Product/2
  [p2] -> Product1/1
  [T2] -> Product1/2
  Product/1 -> Sum1/1
  Product1/1 -> Sum1/2
  Sum1/1 -> T/1  "T"
  [p1] -> Product2/1
  [X2] -> Product3/2
  [p2] -> Product3/1
  Sum2/1 -> X/1  "X"
  Product3/1 -> Sum2/2
  Product2/1 -> Sum2/1
  [X1] -> Product2/2

== system niof_model/GH2/RF System/Subsystem1/Crop Interactio with Climate ==
  C1 : Inport
  C2 : Inport  Port=2
  C3 : Inport  Port=3
  C4 : Inport  Port=4
  Crop2ExtArray{,1..3} (4 alike) : HORTISIM/Other  Functions/Crop2ExtArray  SystemSampleTime=-1  VariantActivationTime=update diagram  Latency=0  AutoFrameSizeCalculation=off
      settings: SourceProductName=Horti Simulator
  Demux : Demux
  Sum : Sum  Inputs=+  CollapseMode=Specified dimension  CollapseDim=2
  Vector Concatenate : Concatenate  NumInputs=4  Mode=Multidimensional array  ConcatenateDimension=2
  Out Bus Element : Outport  PortName=OutBus  Element=HeatVars.QV
  Out Bus Element1 : Outport  PortName=OutBus  Element=HeatVars.QT
  Out Bus Element2 : Outport  PortName=OutBus  Element=A_v
  Out Bus Element3 : Outport  PortName=OutBus  Element=CC
  wires:
  C1/1 -> Crop2ExtArray/1
  C2/1 -> Crop2ExtArray1/1
  C3/1 -> Crop2ExtArray2/1
  C4/1 -> Crop2ExtArray3/1
  Crop2ExtArray3/1 -> Vector Concatenate/4
  Crop2ExtArray2/1 -> Vector Concatenate/3
  Crop2ExtArray1/1 -> Vector Concatenate/2
  Crop2ExtArray/1 -> Vector Concatenate/1
  Vector Concatenate/1 -> Sum/1
  Sum/1 -> Demux/1
  Demux/1 -> Out Bus Element/1
  Demux/2 -> Out Bus Element1/1
  Demux/3 -> Out Bus Element2/1
  Demux/4 -> Out Bus Element3/1

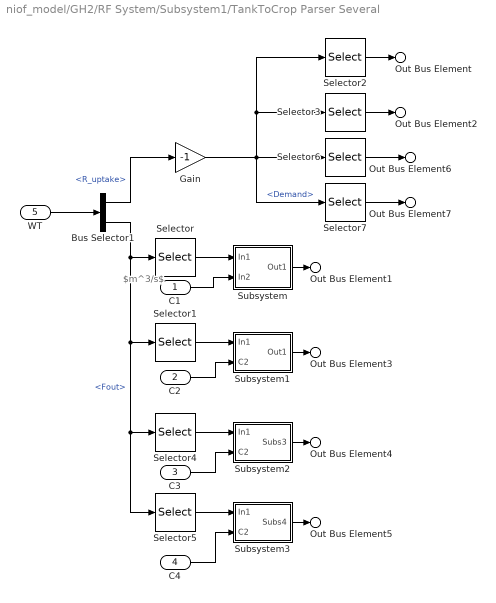
== system niof_model/GH2/RF System/Subsystem1/TankToCrop Parser Several ==
  note: $m^3/s$
  C1 : Inport
  C2 : Inport  Port=2
  C3 : Inport  Port=3
  C4 : Inport  Port=4
  WT : Inport  Port=5
  Bus Selector1 : BusSelector  OutputSignals=R_uptake,Fout
  Gain : Gain  Gain=-1
  Selector : Selector  InputPortWidth=4  IndexOptions=Index vector (dialog)  Indices=[1]  OutputSizes=1
  Selector1 : Selector  InputPortWidth=4  IndexOptions=Index vector (dialog)  Indices=[2]  OutputSizes=1
  Selector2 : Selector  NumberOfDimensions=2  InputPortWidth=2  IndexOptions=Select all,Index vector (dialog)  Indices=[1],1  OutputSizes=1,1
  Selector3 : Selector  NumberOfDimensions=2  InputPortWidth=2  IndexOptions=Select all,Index vector (dialog)  Indices=[2],2  OutputSizes=1,1
  Selector4 : Selector  InputPortWidth=4  IndexOptions=Index vector (dialog)  Indices=[3]  OutputSizes=1
  Selector5 : Selector  InputPortWidth=4  IndexOptions=Index vector (dialog)  Indices=[4]  OutputSizes=1
  Selector6 : Selector  NumberOfDimensions=2  InputPortWidth=2  IndexOptions=Select all,Index vector (dialog)  Indices=[2],3  OutputSizes=1,1
  Selector7 : Selector  NumberOfDimensions=2  InputPortWidth=2  IndexOptions=Select all,Index vector (dialog)  Indices=[2],4  OutputSizes=1,1
  Subsystem : Subsystem
  Subsystem1 : Subsystem
  Subsystem2 : Subsystem
  Subsystem3 : Subsystem
  Out Bus Element1 : Outport  PortName=Subs1  Element=Uptake.Water
  Out Bus Element : Outport  PortName=Subs1  Element=Uptake.Nutrients
  Out Bus Element2 : Outport  Port=2  PortName=Subs2  Element=Uptake.Nutrients
  Out Bus Element3 : Outport  Port=2  PortName=Subs2  Element=Uptake.Water
  Out Bus Element6 : Outport  Port=3  PortName=Subs3  Element=Uptake.Nutrients
  Out Bus Element4 : Outport  Port=3  PortName=Subs3  Element=Uptake.Water
  Out Bus Element7 : Outport  Port=4  PortName=Subs4  Element=Uptake.Nutrients
  Out Bus Element5 : Outport  Port=4  PortName=Subs4  Element=Uptake.Water
  wires:
  WT/1 -> Bus Selector1/1
  Bus Selector1/1 -> Gain/1  "<R_uptake>"
  Gain/1 -> Selector7/1, Selector6/1, Selector3/1, Selector2/1  "<Demand>"
  Selector2/1 -> Out Bus Element/1
  Selector3/1 -> Out Bus Element2/1
  Selector/1 -> Subsystem/1(In1)
  C1/1 -> Subsystem/2(In2)
  Subsystem/1(Out1) -> Out Bus Element1/1
  Selector1/1 -> Subsystem1/1(In1)
  C2/1 -> Subsystem1/2(C2)
  Subsystem1/1(Out1) -> Out Bus Element3/1
  Selector4/1 -> Subsystem2/1(In1)
  C3/1 -> Subsystem2/2(C2)
  Bus Selector1/2 -> Selector5/1, Selector4/1, Selector1/1, Selector/1  "<Fout>"
  Selector5/1 -> Subsystem3/1(In1)
  C4/1 -> Subsystem3/2(C2)
  Subsystem2/1("Subs3 ") -> Out Bus Element4/1
  Subsystem3/1(Subs4) -> Out Bus Element5/1
  Selector6/1 -> Out Bus Element6/1
  Selector7/1 -> Out Bus Element7/1

== system niof_model/GH2/TRAD System/Subsystem1/Crop Interactio with Climate ==
  C1 : Inport
  C2 : Inport  Port=2
  C3 : Inport  Port=3
  C4 : Inport  Port=4
  Crop2ExtArray{,1..3} (4 alike) : HORTISIM/Other  Functions/Crop2ExtArray  SystemSampleTime=-1  VariantActivationTime=update diagram  Latency=0  AutoFrameSizeCalculation=off
      settings: SourceProductName=Horti Simulator
  Demux : Demux
  Sum : Sum  Inputs=+  CollapseMode=Specified dimension  CollapseDim=2
  Vector Concatenate : Concatenate  NumInputs=4  Mode=Multidimensional array  ConcatenateDimension=2
  Out Bus Element : Outport  PortName=OutBus  Element=HeatVars.QV
  Out Bus Element1 : Outport  PortName=OutBus  Element=HeatVars.QT
  Out Bus Element2 : Outport  PortName=OutBus  Element=A_v
  Out Bus Element3 : Outport  PortName=OutBus  Element=CC
  wires:
  C1/1 -> Crop2ExtArray/1
  C2/1 -> Crop2ExtArray1/1
  C3/1 -> Crop2ExtArray2/1
  C4/1 -> Crop2ExtArray3/1
  Crop2ExtArray3/1 -> Vector Concatenate/4
  Crop2ExtArray2/1 -> Vector Concatenate/3
  Crop2ExtArray1/1 -> Vector Concatenate/2
  Crop2ExtArray/1 -> Vector Concatenate/1
  Vector Concatenate/1 -> Sum/1
  Sum/1 -> Demux/1
  Demux/1 -> Out Bus Element/1
  Demux/2 -> Out Bus Element1/1
  Demux/3 -> Out Bus Element2/1
  Demux/4 -> Out Bus Element3/1
